simulink model "hapticsSimBlk_pd"  (Simulink 7.8)
settings: Solver=FixedStepDiscrete  StartTime=0.0  StopTime=100  FixedStep=0.0001  RelTol=1e-3
undefined symbols (not defined in the file or in its folder): DiscIntNeverNeededParam
libraries: vrlib x1, RT x1
settings Model: Creator=Mengchen  LastModifiedBy=z9j7
settings OptimizationCC: InitFltsAndDblsToZero=on
settings DebuggingCC: AlgebraicLoopMsg=error  SaveWithParameterizedLinksMsg=none  FcnCallInpInsideContextMsg=Use local settings  StrictBusMsg=Warning
settings HardwareCC: TargetEndianess=LittleEndian  TargetHWDeviceType=MATLAB Host
settings RTWCC: ProcessScript=grt_make_rtw_hook  CustomHeaderCode="#include \"haptics.h\""  CustomInclude="\"C:\\Program Files\\novint\\HDAL_SDK_1.1.0_Beta\\include\""  TargetLang=C++

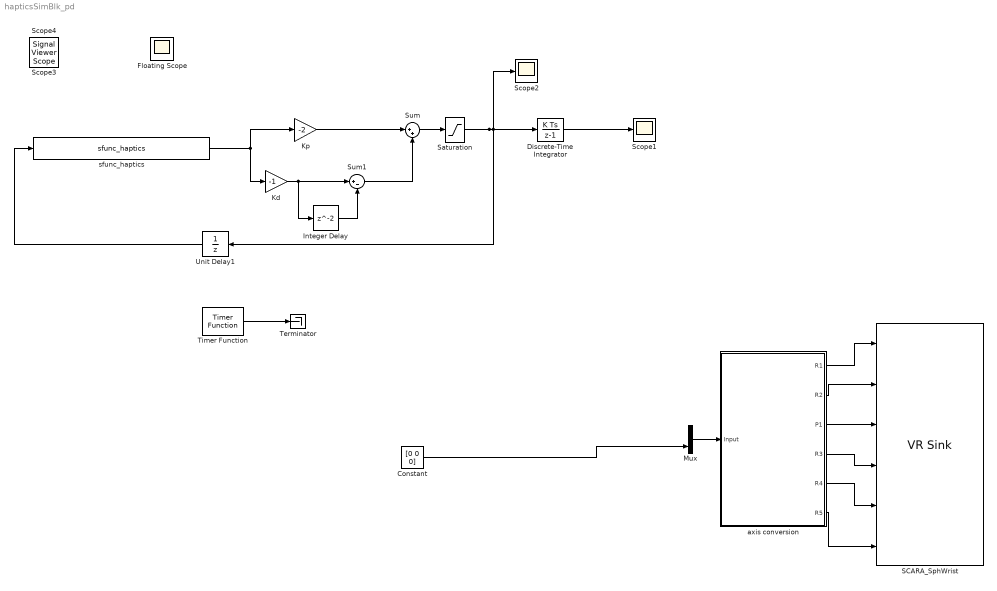
== system hapticsSimBlk_pd ==
  Constant : Constant  Value=[0 0 0]
  Discrete-Time Integrator : DiscreteIntegrator  SampleTime=-1  LimitOutput=on  UpperSaturationLimit=20  LowerSaturationLimit=-20  ICPrevOutput=DiscIntNeverNeededParam  ICPrevScaledInput=DiscIntNeverNeededParam
  Integer Delay : Delay  InputProcessing=Inherited
  Kd : Gain  Gain=-1
  Kp : Gain  Gain=-2
  Mux : Mux  Inputs=2
  SCARA_SphWrist : vrlib/VR Sink  SampleTime=0.1  ViewEnable=on  RemoteChange=off  RemoteView=on  FieldsWritten=R1.rotation.4.1.double#R2.rotation.4.1.double#P1.translation.3.1.double#R3.rotation.4.1.double#R4.rotation.4.1.double#R5.rotation.4.1.double  WorldFileName=ScarawithSphericalWrist.WRL  WorldDescription=SCARA Robot Simulation  AutoView=off  VideoDimensions=[]  AllowVariableSize=off
  Saturation : Saturate  UpperLimit=200  LowerLimit=-200
  Scope1 : Scope
      settings: YMin=-10  YMax=10
  Scope2 : Scope
      settings: YMin=0  YMax=2.75  SaveName=ScopeData2
  Sum : Sum  Inputs=|++
  Sum1 : Sum  Inputs=|+-
  Terminator : Terminator
  Timer Function : RT/Timer Function  step1=0.5  priority1=HIGH  ThPriority1=TIME CRITICAL
  Unit Delay1 : UnitDelay  SampleTime=-1
  axis conversion : Subsystem
  sfunc_haptics : S-Function  FunctionName=sfunc_haptics  EnableBusSupport=off  mask(Legacy Function){SFunctionSpec=void falconPlant(double u1[3], double y1[3]), ShowSpec=on}
      mask prompts: ShowSpec "Display function specification"
      mask help:
      | This block allows you to call the legacy functions specified by the following Legacy Code Tool definition:
      | def.SFunctionName = 'sfunc_haptics';
      | def.OutputFcnSpec = 'void falconPlant(double u1[3], double y1[3])';
      | def.StartFcnSpec = 'createHaptics()';
      | def.TerminateFcnSpec = 'deleteHaptics()';
      | def.HeaderFiles = {'haptics.h'};
      | def.SourceFiles = {'haptics.cpp'};
      | def.HostLibFiles = {'hdl.lib'};
      | def.TargetLibFiles = {'hdl.lib'};
      | def.IncPaths = {'C:\Documents and Settings\z9j7\Desktop\HDAL_SDK_2.1.3\include'};
      | def.LibPaths = {'C:\Documents and Settings\z9j7\Desktop\HDAL_SDK_2.1.3\lib'};
      | def.Options.useTlcWithAccel = false;
      | def.Options.language = 'C++';
      mask Help: <p>This block was generated automatically by the Legacy Code Tool. For detailed help on this tool, call<a href="matlab:legacy_code('help')"> legacy_code('help')</a>.</p>
      mask CallbackString:
      | |if strcmp(get_param(gcbh, 'ShowSpec'), 'on')
      |   set_param(gcbh, 'MaskDisplay', sprintf('fprintf(''%s'');', get_param(gcbh, 'SFunctionSpec')));
      | else
      |   set_param(gcbh, 'MaskDisplay', sprintf('fprintf(''%s'');', get_param(gcbh, 'FunctionName')));
      | end
      mask Display: fprintf('void falconPlant(double u1[3], double y1[3])');
  Floating Scope : Scope
      settings: Floating=on  SaveName=ScopeData3
  Scope3 : SignalViewerScope  IOType=viewer  RefreshTime=0.035000
  Scope4 : SignalViewerScope  IOType=viewer  RefreshTime=0.035000
  wires:
  sfunc_haptics/1 -> Kd/1, Kp/1
  Kp/1 -> Sum/1
  Sum/1 -> Saturation/1
  Saturation/1 -> Unit Delay1/1, Scope2/1, Discrete-Time Integrator/1
  Kd/1 -> Sum1/1, Integer Delay/1
  Unit Delay1/1 -> sfunc_haptics/1
  Sum1/1 -> Sum/2
  Integer Delay/1 -> Sum1/2
  Timer Function/1 -> Terminator/1
  axis conversion/1(R1) -> SCARA_SphWrist/1
  axis conversion/2(R2) -> SCARA_SphWrist/2
  axis conversion/3(P1) -> SCARA_SphWrist/3
  axis conversion/4(R3) -> SCARA_SphWrist/4
  axis conversion/5(R4) -> SCARA_SphWrist/5
  axis conversion/6(R5) -> SCARA_SphWrist/6
  Mux/1 -> axis conversion/1(Input)
  Constant/1 -> Mux/2
  Discrete-Time Integrator/1 -> Scope1/1

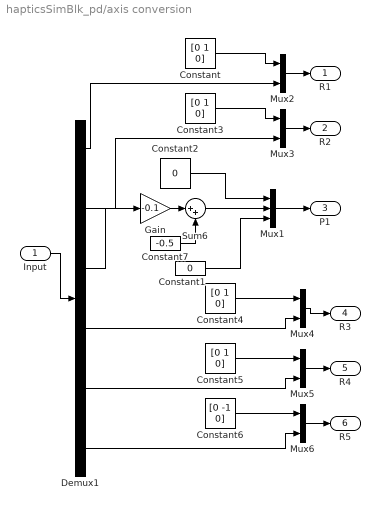
== system hapticsSimBlk_pd/axis conversion ==
  Input : Inport
  Constant{,3..5} (4 alike) : Constant  Value=[0 1 0]
  Constant1 : Constant  Value=0
  Constant2 : Constant  Value=0
  Constant6 : Constant  Value=[0 -1 0]
  Constant7 : Constant  Value=-0.5
  Demux1 : Demux  Outputs=6
  Gain : Gain  Gain=-0.1
  Mux1 : Mux  Inputs=3
  Mux{2..6} (5 alike) : Mux  Inputs=2
  Sum6 : Sum  Inputs=|++
  R1 : Outport
  R2 : Outport  Port=2
  P1 : Outport  Port=3
  R3 : Outport  Port=4
  R4 : Outport  Port=5
  R5 : Outport  Port=6
  wires:
  Sum6/1 -> Mux1/2
  Constant2/1 -> Mux1/1
  Demux1/6 -> Mux6/2
  Demux1/4 -> Mux4/2
  Demux1/3 -> Gain/1
  Demux1/2 -> Mux3/2
  Constant1/1 -> Mux1/3
  Mux1/1 -> P1/1
  Constant7/1 -> Sum6/2
  Gain/1 -> Sum6/1
  Demux1/5 -> Mux5/2
  Demux1/1 -> Mux2/2
  Mux6/1 -> R5/1
  Mux5/1 -> R4/1
  Mux4/1 -> R3/1
  Input/1 -> Demux1/1
  Mux3/1 -> R2/1
  Mux2/1 -> R1/1
  Constant6/1 -> Mux6/1
  Constant5/1 -> Mux5/1
  Constant4/1 -> Mux4/1
  Constant3/1 -> Mux3/1
  Constant/1 -> Mux2/1
